simulink model "DCC_DTC_v3"  (R2023b)
settings: Solver=FixedStepDiscrete  StartTime=0.0  StopTime=0.4  MaxStep=1e-  RelTol=1e-6
undefined symbols (not defined in the file): DiscIntNeverNeededParam
libraries: spsDCVoltageSourceLib x1, spsGroundLib x1, spsPermanentMagnetSynchronousMachineLib x1, simulink x1, spsThreePhaseVIMeasurementLib x1, spsUniversalBridgeLib x1, sps_lib x1
settings Model: Creator=rainy  LastModifiedBy=rainy
settings DataIOCC: ReturnWorkspaceOutputs=off

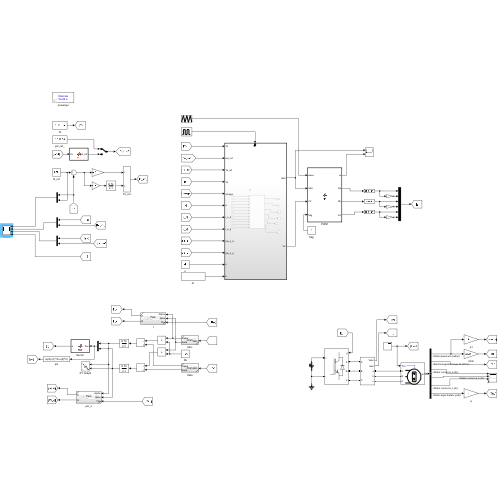
[thumbnail: Simulink's stored preview of the top-level diagram]
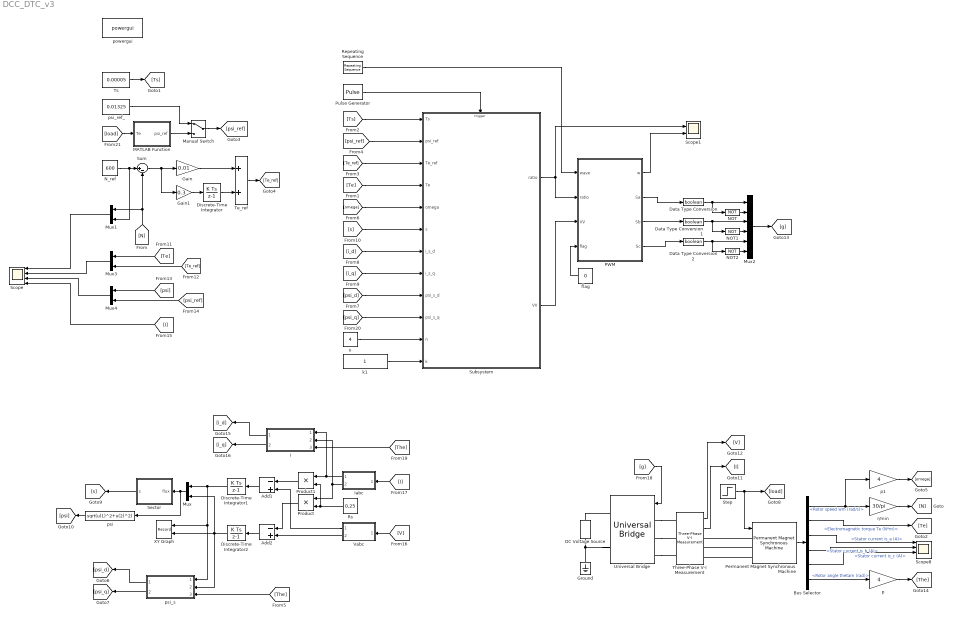
== system DCC_DTC_v3 ==
  Add1 : Sum  Inputs=-+
  Add2 : Sum  Inputs=-+
  Bus Selector : BusSelector  OutputSignals=Rotor speed wm (rad/s),Electromagnetic torque Te (N*m),Stator current is_a (A),Stator current is_b (A),Stator current is_c (A),Rotor angle thetam (rad)
  DC Voltage Source : spsDCVoltageSourceLib/DC Voltage Source  Amplitude=24  Measurements=Voltage
  Data Type Conversion : DataTypeConversion  OutDataTypeStr=boolean  SaturateOnIntegerOverflow=off  RndMeth=Floor
  Data Type Conversion1 : DataTypeConversion  OutDataTypeStr=boolean  SaturateOnIntegerOverflow=off  RndMeth=Floor
  Data Type Conversion2 : DataTypeConversion  OutDataTypeStr=boolean  SaturateOnIntegerOverflow=off  RndMeth=Floor
  Discrete-Time Integrator : DiscreteIntegrator  SampleTime=-1  ICPrevOutput=DiscIntNeverNeededParam  ICPrevScaledInput=DiscIntNeverNeededParam
  Discrete-Time Integrator1 : DiscreteIntegrator  SampleTime=-1  ICPrevOutput=DiscIntNeverNeededParam  ICPrevScaledInput=DiscIntNeverNeededParam
  Discrete-Time Integrator2 : DiscreteIntegrator  SampleTime=-1  ICPrevOutput=DiscIntNeverNeededParam  ICPrevScaledInput=DiscIntNeverNeededParam
  Gain : Gain  Gain=0.01
  Gain1 : Gain  Gain=0.3
  Ground : spsGroundLib/Ground  LConnTagsString=a
  I : Subsystem  ReferencedSubsystem=Park
  Iabc : Subsystem  ReferencedSubsystem=Clark
  MATLAB Function : MATLAB Function  TreatAsAtomicUnit=on
  Manual Switch : ManualSwitch
  Mux{,1,3..4} (4 alike) : Mux  Inputs=2
  Mux2 : Mux  Inputs=6
  NOT : Logic  Operator=NOT  IconShape=distinctive  AllPortsSameDT=off  OutDataTypeStr=boolean
  NOT1 : Logic  Operator=NOT  IconShape=distinctive  AllPortsSameDT=off  OutDataTypeStr=boolean
  NOT2 : Logic  Operator=NOT  IconShape=distinctive  AllPortsSameDT=off  OutDataTypeStr=boolean
  N_ref : Constant  Value=600
  PWM : MATLAB Function  TreatAsAtomicUnit=on
  Permanent Magnet Synchronous Machine : spsPermanentMagnetSynchronousMachineLib/Permanent Magnet Synchronous Machine  NbPhases=3  FluxDistribution=Sinusoidal  RotorType=Round  MechanicalLoad=Torque Tm  PresetModel=No  ShowDetailedParameters=on  MeasurementBus=off  Resistance=0.25  Inductance=8.5e-3  dqInductances=[0.0133 0.0147]  La=0.0005  MachineConstant=Flux linkage established by magnets (V.s)  Flux=0.01325  VoltageCst=9.6131  TorqueCst=0.0795  Flat=120  Mechanical=[0.00003 0 4 0]  PolePairs=2  InitialConditions=[0 0 0 0]  InitialConditions5ph=[0 0 0 0 0 0]  RefAngle=Aligned with phase A axis (original Park)  IterativeDiscreteModel=Trapezoidal non iterative  TsBlock=-1  TsPowergui=0
  Product : Product
  Product1 : Product
  Pulse Generator : DiscretePulseGenerator  PulseType=Time based  Period=0.00005
  Repeating Sequence : simulink/Sources/Repeating Sequence  rep_seq_t=[0 0.000025 0.00005]  rep_seq_y=[0 1 0]
  Rs : Constant  Value=0.25
  Scope : Scope  NumInputPorts=4
  Scope1 : Scope  NumInputPorts=2
  Scope8 : Scope  NumInputPorts=4
  Sector : MATLAB Function  TreatAsAtomicUnit=on
  Step : Step  Time=0.2  After=0.5  SampleTime=0
  Subsystem : Subsystem
  Sum : Sum  Inputs=|+-
  Te_ref : Sum
  Three-Phase V-I Measurement : spsThreePhaseVIMeasurementLib/Three-Phase V-I Measurement  VoltageMeasurement=phase-to-ground  SetLabelV=off  LabelV=Vabc  Vpu=off  VpuLL=off  CurrentMeasurement=yes  SetLabelI=off  LabelI=Iabc  Ipu=off  Pbase=100e6  Vbase=500e3  OutputType=Complex  PhasorSimulation=off  PSBequivalent=0
  Ts : Constant  Value=0.00005
  Universal Bridge : spsUniversalBridgeLib/Universal Bridge  Arms=3  SnubberResistance=1e5  SnubberCapacitance=inf  Device=IGBT / Diodes  Ron=1e-3  Lon=0  ForwardVoltages="[  0  0  ]"  ForwardVoltage=0  GTOparameters=[ 10e-6 , 20e-6 ]  IGBTparameters=[ 1e-6 , 2e-6 ]  Measurements=None  Measurements_2=None  converterType=Rectifier
  Vabc : Subsystem  ReferencedSubsystem=Clark
  XY Graph : Record  FileSettingsInternal="{\"entries\":[{\"content\":{\"excelSettings\":{\"content\":{},\"type\":\"Streamout.ExcelSettings\"}},\"type\":\"Streamout.FileSettingStorage\",\"uuid\":\"\"}],\"packageUris\":[\"http:\\/\\/schema.mathworks.com\\/mf0\\/streamout_blocks\\/R2020a\"],\"version\":\"1.0\"}"  Layout=[1 1]  SignalsInternal="{\"entries\":[{\"content\":{\"signals\":[{\"content\":{\"blockPath\":[],\"dimensions\":[1],\"domain\":\"\",\"lineColor\":\"#a2142f\",\"plots\":[1],\"port\":1,\"sid\":[\"\"],\"signalID\":7296,\"signalName\":\"Discrete-Time\\nIntegrator1\"},\"type\":\"RecordBlkView.Signal\",\"uuid\":\"\"},{\"content\":{\"blockPath\":[],\"dimensions\":[1],\"domain\":\"\",\"lineColor\":\"#139fff\",\"plots\":[1],\"port\":2,\"sid\":[\"\"],\"signalID\":7300,\"signalName\":\"Discrete-Time\\nIntegrator2\"},\"type\":\"RecordBlkView.Signal\",\"uuid\":\"\"}]},\"type\":\"RecordBlkView.InputSignals\",\"uuid\":\"\"}],\"packageUris\":[\"http:\\/\\/schema.mathworks.com\\/mf0\\/streamout_blocks\\/R2020a\"],\"version\":\"1.0\"}"  VisualizationBindings="{\"xyplotplugin\":{\"info\":[{\"series\":[{\"bindingParametersList\":[{\"parameter\":\"X-Axis\",\"signalID\":7296,\"signalName\":\"Discrete-Time\\nIntegrator1\"},{\"parameter\":\"Y-Axis\",\"signalID\":7300,\"signalName\":\"Discrete-Time\\nIntegrator2\"}],\"seriesID\":44098}],\"subplotID\":1}]}}"  CompatibilityTag=XY  st=-1
  flag : Constant  Value=0
  k1 : Constant
  n : Constant  Value=4
  p : Gain  Gain=4
  p1 : Gain  Gain=4
  powergui : sps_lib/powergui  Priority=1  SimulationMode=Discrete  SampleTime=5e-6  frequency=60  Iterations=50  frequencyindice=0  Pbase=100e6  ErrMax=1e-4  UnitsV=kV  UnitsW=MW  buscounter=0  FunctionMessages=off  echomessages=off  EnableUseOfTLC=off  CurrentSourceSwitches=off  DisableSnubberDevices=off  DisableRonSwitches=off  DisableVfSwitches=off  DisplayEquations=off  AutomaticDiscreteSolvers=off  SolverType=Tustin/Backward Euler (TBE)  Interpol=off  ExternalGateDelay=off  methode=off  Ts=100  x0status=blocks  SPID=on  SwTol=0  HookPort=off  NonlinearTolerance=1e-4  nMaxIteration=100  ContinueOnMaxIteration=off  RestoreLinks=warning  ResistiveCurrentMeasurement=off  Frange=[0:2:500]  Ylog=off  Xlog=on  ShowGrid=off  save=off  variable=ZData  structure=0  ZoomFFT=off  StartTime=0.0  cycles=1  DisplayStyle=1  fundamental=60  FreqAxis=off  MaxFrequency=1000  frequencyindicesteady=1  RmsSteady=1  display=off
  psi : Fcn  Expr=sqrt(u(1)^2+u(2)^2)
  psi_ref_ : Constant  Value=0.01325
  psi_s : Subsystem  ReferencedSubsystem=Park
  r/min : Gain  Gain=30/pi
  wires:
  N_ref/1 -> Mux1/2, Sum/1
  Sum/1 -> Gain/1, Gain1/1
  Gain1/1 -> Discrete-Time Integrator/1
  Gain/1 -> Te_ref/1
  Permanent Magnet Synchronous Machine/1 -> Bus Selector/1
  Bus Selector/1 -> p1/1, r/min/1  "<Rotor speed wm (rad/s)>"
  r/min/1 -> [N]
  [N] -> Sum/2, Mux1/1
  NOT1/1 -> Mux2/4
  Data Type Conversion2/1 -> NOT2/1, Mux2/5
  NOT2/1 -> Mux2/6
  Data Type Conversion/1 -> NOT/1, Mux2/1
  NOT/1 -> Mux2/2
  Data Type Conversion1/1 -> NOT1/1, Mux2/3
  Iabc/1 -> I/1, Product1/1
  Iabc/2 -> Product/1, I/2
  Rs/1 -> Product/2, Product1/2
  Product1/1 -> Add1/1
  Vabc/1 -> Add1/2
  Product/1 -> Add2/1
  Vabc/2 -> Add2/2
  Add2/1 -> Discrete-Time Integrator2/1
  Add1/1 -> Discrete-Time Integrator1/1
  Ts/1 -> [Ts]
  Mux/1 -> psi/1, Sector/1(flux)
  Bus Selector/2 -> [Te]  "<Electromagnetic torque Te (N*m)>"
  [Te] -> Subsystem/4(Te)
  Three-Phase V-I Measurement/2 -> [I]
  Discrete-Time Integrator/1 -> Te_ref/2
  PWM/4(Sc) -> Data Type Conversion2/1
  PWM/3(Sb) -> Data Type Conversion1/1
  PWM/2(Sa) -> Data Type Conversion/1
  [Ts] -> Subsystem/1(Ts)
  [psi_ref] -> Subsystem/2(psi_ref)
  Repeating Sequence/1 -> PWM/1(wave)
  Pulse Generator/1 -> Subsystem/Trigger
  n/1 -> Subsystem/11(n)
  flag/1 -> PWM/4(flag)
  Bus Selector/3 -> Scope8/1  "<Stator current is_a (A)>"
  Bus Selector/4 -> Scope8/2  "<Stator current is_b (A)>"
  Bus Selector/5 -> Scope8/3  "<Stator current is_c (A)>"
  Step/1 -> [load], Permanent Magnet Synchronous Machine/1
  Subsystem/1(ratio) -> Scope1/1, PWM/2(ratio)
  Subsystem/2(VV) -> PWM/3(VV)
  Te_ref/1 -> [Te_ref]
  [Te_ref] -> Subsystem/3(Te_ref)
  [omega] -> Subsystem/5(omega)
  [i_d] -> Subsystem/7(i_s_d)
  [i_q] -> Subsystem/8(i_s_q)
  Sector/1(s) -> [s]
  [s] -> Subsystem/6(s)
  PWM/1(w) -> Scope1/2
  psi/1 -> [psi]
  Mux1/1 -> Scope/1
  Mux3/1 -> Scope/2
  Mux4/1 -> Scope/3
  [I] -> Scope/4
  [Te] -> Mux3/1
  [psi] -> Mux4/1
  [Te_ref] -> Mux3/2
  [psi_ref] -> Mux4/2
  Three-Phase V-I Measurement/1 -> [V]
  [I] -> Iabc/1
  [V] -> Vabc/1
  Mux2/1 -> [g]
  [g] -> Universal Bridge/1
  Bus Selector/6 -> p/1  "<Rotor angle thetam (rad)>"
  p/1 -> [The]
  [The] -> I/3
  I/2 -> [i_q]
  I/1 -> [i_d]
  p1/1 -> [omega]
  k1/1 -> Subsystem/12(k)
  psi_s/1 -> [psi_d]
  Discrete-Time Integrator1/1 -> XY Graph/1, psi_s/1, Mux/1
  psi_s/2 -> [psi_q]
  [The] -> psi_s/3
  Discrete-Time Integrator2/1 -> psi_s/2, XY Graph/2, Mux/2
  [psi_q] -> Subsystem/10(psi_s_q)
  [psi_d] -> Subsystem/9(psi_s_d)
  [load] -> MATLAB Function/1(Te)
  psi_ref_/1 -> Manual Switch/1
  MATLAB Function/1(psi_ref) -> Manual Switch/2
  Manual Switch/1 -> [psi_ref]
  connections:
  Universal Bridge/RConn2 -- DC Voltage Source/LConn1 -- Ground/LConn1
  Permanent Magnet Synchronous Machine/LConn2 -- Three-Phase V-I Measurement/RConn2
  Permanent Magnet Synchronous Machine/LConn1 -- Three-Phase V-I Measurement/RConn1
  Universal Bridge/LConn3 -- Three-Phase V-I Measurement/LConn3
  Universal Bridge/LConn1 -- Three-Phase V-I Measurement/LConn1
  Universal Bridge/LConn2 -- Three-Phase V-I Measurement/LConn2
  DC Voltage Source/RConn1 -- Universal Bridge/RConn1
  Permanent Magnet Synchronous Machine/LConn3 -- Three-Phase V-I Measurement/RConn3

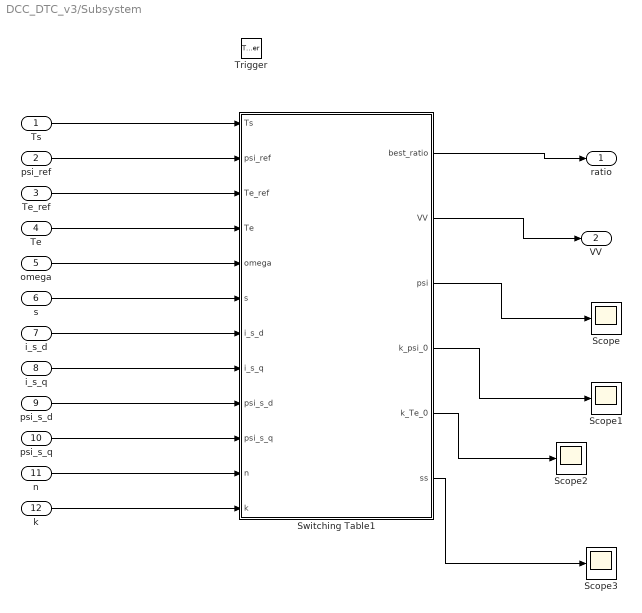
== system DCC_DTC_v3/Subsystem ==
  Ts : Inport
  psi_ref : Inport  Port=2
  Te_ref : Inport  Port=3
  Te : Inport  Port=4
  omega : Inport  Port=5
  s : Inport  Port=6
  i_s_d : Inport  Port=7
  i_s_q : Inport  Port=8
  psi_s_d : Inport  Port=9
  psi_s_q : Inport  Port=10
  n : Inport  Port=11
  k : Inport  Port=12
  Trigger : TriggerPort  VariantControl=(inherit)  PortDimensions=1
  Scope{,1..3} (4 alike) : Scope
  Switching Table1 : MATLAB Function  TreatAsAtomicUnit=on
  ratio : Outport
  VV : Outport  Port=2
  wires:
  Ts/1 -> Switching Table1/1(Ts)
  psi_ref/1 -> Switching Table1/2(psi_ref)
  Te_ref/1 -> Switching Table1/3(Te_ref)
  Te/1 -> Switching Table1/4(Te)
  omega/1 -> Switching Table1/5(omega)
  s/1 -> Switching Table1/6(s)
  i_s_q/1 -> Switching Table1/8(i_s_q)
  Switching Table1/1(best_ratio) -> ratio/1
  k/1 -> Switching Table1/12(k)
  n/1 -> Switching Table1/11(n)
  Switching Table1/2(VV) -> VV/1
  i_s_d/1 -> Switching Table1/7(i_s_d)
  Switching Table1/3(psi) -> Scope/1
  psi_s_q/1 -> Switching Table1/10(psi_s_q)
  psi_s_d/1 -> Switching Table1/9(psi_s_d)
  Switching Table1/4(k_psi_0) -> Scope1/1
  Switching Table1/5(k_Te_0) -> Scope2/1
  Switching Table1/6(ss) -> Scope3/1

== matlab function DCC_DTC_v3/Subsystem/Switching Table1 ==
  data: best_ratio output; Ts input; psi_ref input; Te_ref input; Te input; VV output; omega input; s input; i_s_d input; i_s_q input; psi_s_d input; psi_s_q input; n input; k input; psi output; k_psi_0 output; k_Te_0 output; ss output
function [best_ratio, VV, psi, k_psi_0, k_Te_0, ss]= fcn(Ts, psi_ref, Te_ref, Te, omega, s, i_s_d, i_s_q, psi_s_d, psi_s_q, n, k)

% 给定的参数值
p = 4;
R_s = 0.25;
L_d = 0.0005;
L_q = 0.0005;
V = 24;
psi_f = 0.01325;

psi_r = psi_f + 1i*0;
psi_s_d = L_d*i_s_d + psi_f;
psi_s_q = L_q*i_s_q;

i_s = i_s_d + 1i*i_s_q;
psi_s = psi_s_d + 1i*psi_s_q;


% 计算零电压矢量下变化率
psi = sqrt(psi_s_d^2 +psi_s_q^2);
k_psi_0 = -R_s/psi*real(psi_s'*i_s); % 零电压矢量时磁链变化率
% k_psi_1 = 1/psi*real(psi_s'*u_s) + k_psi_0; % 非零电压矢量时磁链变化率

k_Te_0 = -3/2*p*(1/L_q-1/L_d)*omega*real(psi_s^2) + ...
    3/4*p*R_s*(1/L_d^2-1/L_q^2)*imag(psi_s^2) - ...
    3/2*p/L_d*(R_s/L_d*imag(psi_s*psi_r) + omega*real(psi_s*psi_r)); % 零电压矢量时转矩变化率
ss = psi_s*psi_r;
% k_Te_1 = 3/2*p*(1/L_q-1/L_d)*imag(u_s*psi_s) + 3/2*p/L_d*imag(u_s*psi_r) + k_Te_0;  % 非零电压矢量时转矩变化率



% 选择电压矢量
Te1 = Te + k_Te_0*Ts;
psi1 = psi + k_psi_0*Ts;

if(Te_ref > Te)
    if(psi_ref > psi)
        VV = s+1;
    else
        VV = s+2;
    end
else
    if(psi_ref > psi)
        VV = s-1;
    else
        VV = s-2;
    end
end

if(VV < 1)
    VV = VV+6;
end
if(VV > 6)
    VV = VV-6;
end


% MPTC
u_s = cos(pi/6*(VV-1))*V + 1i*sin(pi/6*(VV-1))*V;
k_psi_1 = 1/psi*real(psi_s'*u_s) + k_psi_0; % 非零电压矢量时磁链变化率
k_Te_1 = 3/2*p*(1/L_q-1/L_d)*imag(u_s*psi_s) + 3/2*p/L_d*imag(u_s*psi_r) + k_Te_0;  % 非零电压矢量时转矩变化率

g_min = Inf;
best_ratio = 1;

d_Te = 0;
d_psi = 0;

for i=1:n+1
    ratio = (i-1)*1/n;

    Te1_ = Te + Ts*ratio*k_Te_1 + Ts*(1-ratio)*k_Te_0;
    psi_s1 = psi_s + Ts*ratio*k_psi_1 + Ts*(1-ratio)*k_psi_0;
    
    d_Te = abs(Te_ref - Te1_);
    d_psi = k*abs(psi_ref - abs(psi_s1));

    g = d_Te + d_psi;

    if(g < g_min)
        g_min = g;
        best_ratio =ratio;
    end
end

== matlab function DCC_DTC_v3/MATLAB Function ==
  data: Te input; psi_ref output
function psi_ref = fcn(Te)

p = 2;
R_s = 4.765;
L_d = 0.0133;
L_q = 0.0147;
V = 300;
psi_f = 0.1848;

psi_ref = sqrt(psi_f^2 + ((2*L_q)/(3*p*psi_f))^2);

== matlab function DCC_DTC_v3/Sector ==
  data: flux input; s output
function s = fcn(flux)

% 将\psi_{\aplha}和\psi_{\beta}分解为三相
a1 = flux(1);
b1 = flux(1)*(-0.5) + sqrt(3)/2*flux(2);
c1 = flux(1)*(-0.5) - sqrt(3)/2*flux(2);

% a1 > 0，有扇区126
% b1 > 0，有扇区234
% c1 > 0，有扇区456
% n为a1 b1 c1中>0的个数，0 < n < 3
% 
% a b c | s
%-------|---
% 1 1 0 | 2
% 1 0 1 | 6
% 1 0 0 | 1
% 0 1 1 | 4
% 0 1 0 | 3
% 0 0 1 | 5

if(flux(2) == 0)
    N = 4;
else
    if(a1 > 0)
        a = 1;
    else
        a = 0;
    end
    
    if(b1 > 0)
        b = 1;
    else
        b = 0;
    end
    
    if(c1 > 0)
        c = 1;
    else
        c = 0;
    end
    
    N = 4*a+2*b+c;
end

% if(N==0 || N==7)
%     N = 4;
% end

Sector_table=[5 3 4 1 6 2];

s = Sector_table(N);

== matlab function DCC_DTC_v3/PWM ==
  data: w output; wave input; ratio input; VV input; Sa output; Sb output; Sc output; flag input
function [w, Sa, Sb, Sc] = fcn(wave, ratio, VV, flag)

sw = [1 0 0; 1 1 0; 0 1 0; 0 1 1; 0 0 1; 1 0 1];

if(VV<1 || VV>6)
    VV = 1;
end

if(wave >= 1 - ratio || flag == 0)
    Sa= sw(VV, 1);
    Sb= sw(VV, 2);
    Sc= sw(VV, 3);
    w = 1;
else
    Sa = 0;
    Sb = 0;
    Sc = 0;
    w = 0;
end
